simulink model "BMS_MCU_CODE"  (R2025b)
settings: Solver=FixedStepAuto  StartTime=0.0  StopTime=10  MaxStep=.01  RelTol=1e-3  EnableMultiTasking=on
PreLoadFcn:
  | %setup_sil;
  | setup_pil;
InitFcn:
  | battery_init;
  | Full_Charge_Volt=4.2; % unit volts
  | Cutoff_Volt=3; % unit volts
  | Delta=.02;
  | ContactorTime=20;
  | ContactorTimeOut=100;
  | High_TempLim=333;
  | Low_TempLim=253;
  | Sensor_Fault_Treshold=.02;
  | CurrentTimeout=1;
  | Allowed_Delta=.04;
  | Bal_On_Time=30;
  | Bal_Off_Time=5;
  | BalNotAct_Time=10;
values from neighbouring files (symbols this model uses):
  bonka_R0 = [ ... (first row only)    [battery_init.m]
  bonka_SOC = [0, 0.1, 0.2, 0.3, 0.4, 0.5, 0.6, 0.7, 0.8, 0.9, 1.0]    [battery_init.m]
  bonka_T = [263.15, 273.15, 298.15, 313.15, 328.15]    [battery_init.m]
  Capacity = 5.200    (= 5.2)    [MCU.m]
  Charge_Rate = 1    [battery_init.m]
  Discharge_Rate = -1    [battery_init.m]
undefined symbols (not defined in the file or in its folder): DiscIntNeverNeededParam
libraries: simulink x30
settings Model: DataDictionary=Needed_Buses.sldd  STM32="{\"DigitalPortWrite\":[{\"ID\":\"MCU_CODE:12\"},{\"ID\":\"MCU_CODE_Copy:132\"},{\"ID\":\"BMS_PIL_Wrapper:132\"}],\"DigitalPortRead\":[{\"ID\":\"MCU_CODE_Copy:131\"},{\"ID\":\"BMS_PIL_Wrapper:131\"}]}"  SILPILSystemUnderTest=refmodels  CodeVerificationMode=processor-in-the-loop (pil)  Creator=Odonata-KJ  LastModifiedBy=Odonata-KJ
settings DataIOCC: SaveOutput=off  SaveTime=off
settings OptimizationCC: DefaultParameterBehavior=Inlined  EnhancedBackFolding=on  PassReuseOutputArgsAs=Individual arguments  ZeroExternalMemoryAtStartup=off  ZeroInternalMemoryAtStartup=off  MaxStackSize=512  OptimizeBlockOrder=speed  DifferentSizesBufferReuse=on  OptimizationCustomize=off  EfficientTunableParamExpr=on
settings DebuggingCC: ParameterTunabilityLossMsg=error  SFUnexpectedBacktrackingDiag=warning  SFNoUnconditionalDefaultTransitionDiag=warning  UnderSpecifiedDimensionMsg=warning
settings HardwareCC: ProdBitPerPointer=32.0  ProdBitPerSizeT=32.0  ProdBitPerPtrDiffT=32.0  ProdLargestAtomicInteger=Long  ProdLargestAtomicFloat=Double  ProdWordSize=32.0  ProdLongLongMode=on  ProdHWDeviceType=ARM Compatible->ARM Cortex-M  TargetLargestAtomicInteger=Long  TargetLargestAtomicFloat=Double  TargetIntDivRoundTo=Zero  TargetEndianess=LittleEndian  TargetHWDeviceType=ARM Compatible->ARM Cortex-M
settings SFSimCC: MATLABDynamicMemAlloc=off
settings RTWCC: SystemTargetFile=ert.tlc  HardwareBoard=STM32F4xx Based  TemplateMakefile=ert_default_tmf  GenerateReport=on  Toolchain=GNU Tools for ARM Embedded Processors  BuildConfiguration=Debug  LaunchReport=on  PortableWordSizes=on  Description=Embedded Coder
settings CodeAppCC: ForceParamTrailComments=on  IgnoreCustomStorageClasses=off  OperatorAnnotations=on  SimulinkDataObjDesc=on  SFDataObjDesc=on  InsertBlockDesc=on  EnableCustomComments=on
settings ERTTargetCC: ExtModeTransport=3.0  ExtModeStaticAlloc=on  ExtModeStaticAllocSize=2048.0  ExtModeMexFile=ext_xcp  ExtModeIntrfLevel=Level2 - Open  TargetLangStandard=C99 (ISO)

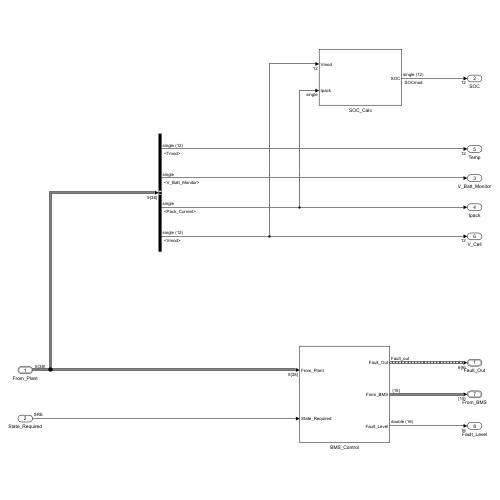
[thumbnail: Simulink's stored preview of the top-level diagram]
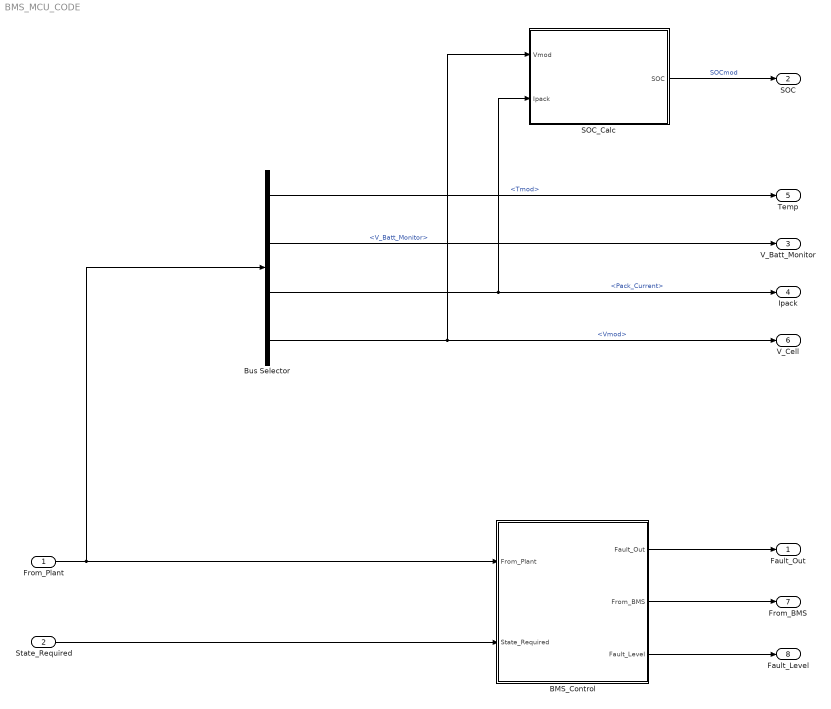
== system BMS_MCU_CODE ==
  From_Plant : Inport  OutDataTypeStr=Bus: From_Plant
  State_Required : Inport  Port=2  OutDataTypeStr=Enum: SRE
  BMS_Control : Subsystem
  Bus Selector : BusSelector  OutputSignals=Tmod,V_Batt_Monitor,Pack_Current,Vmod
  SOC_Calc : Subsystem
  Fault_Out : Outport  OutDataTypeStr=Bus: Fault_out
  SOC : Outport  Port=2
  V_Batt_Monitor : Outport  Port=3
  Ipack : Outport  Port=4
  Temp : Outport  Port=5
  V_Cell : Outport  Port=6
  From_BMS : Outport  Port=7  OutDataTypeStr=Bus: From_BMS
  Fault_Level : Outport  Port=8
  wires:
  From_Plant/1 -> Bus Selector/1, BMS_Control/1(From_Plant)
  BMS_Control/1(Fault_Out) -> Fault_Out/1
  SOC_Calc/1(SOC) -> SOC/1  "SOCmod"
  Bus Selector/1 -> Temp/1  "<Tmod>"
  Bus Selector/3 -> SOC_Calc/2(Ipack), Ipack/1  "<Pack_Current>"
  Bus Selector/4 -> SOC_Calc/1(Vmod), V_Cell/1  "<Vmod>"
  State_Required/1 -> BMS_Control/2(State_Required)
  BMS_Control/2(From_BMS) -> From_BMS/1
  BMS_Control/3(Fault_Level) -> Fault_Level/1
  Bus Selector/2 -> V_Batt_Monitor/1  "<V_Batt_Monitor>"

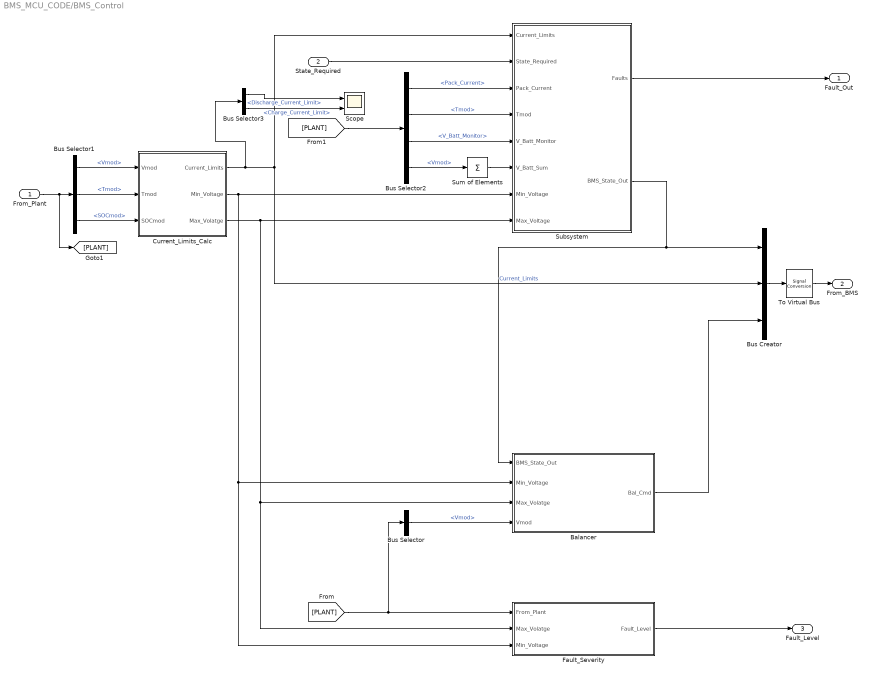
== system BMS_MCU_CODE/BMS_Control ==
  From_Plant : Inport
  State_Required : Inport  Port=2
  Balancer : Subsystem
  Bus Creator : BusCreator  Inputs=3
  Bus Selector : BusSelector  OutputSignals=Vmod
  Bus Selector1 : BusSelector  OutputSignals=Vmod,Tmod,SOCmod
  Bus Selector2 : BusSelector  OutputSignals=Pack_Current,Tmod,V_Batt_Monitor,Vmod
  Bus Selector3 : BusSelector  OutputSignals=Discharge_Current_Limit,Charge_Current_Limit
  Current_Limits_Calc : Subsystem
  Fault_Severity : Subsystem
  Scope : Scope  NumInputPorts=2
  Subsystem : Subsystem
  Sum of Elements : Sum  Inputs=+
  To Virtual Bus : SignalConversion  ConversionOutput=Virtual bus  OverrideOpt=off
  Fault_Out : Outport
  From_BMS : Outport  Port=2  OutDataTypeStr=Bus: From_BMS
  Fault_Level : Outport  Port=3
  wires:
  Bus Selector1/2 -> Current_Limits_Calc/2(Tmod)  "<Tmod>"
  Subsystem/1(Faults) -> Fault_Out/1
  [PLANT] -> Bus Selector2/1
  State_Required/1 -> Subsystem/2(State_Required)
  Current_Limits_Calc/1(Current_Limits) -> Bus Selector3/1, Bus Creator/2, Subsystem/1(Current_Limits)  "Current_Limits"
  Bus Selector1/1 -> Current_Limits_Calc/1(Vmod)  "<Vmod>"
  From_Plant/1 -> Bus Selector1/1, [PLANT]
  Bus Selector2/1 -> Subsystem/3(Pack_Current)  "<Pack_Current>"
  Bus Selector2/2 -> Subsystem/4(Tmod)  "<Tmod>"
  Bus Selector2/3 -> Subsystem/5(V_Batt_Monitor)  "<V_Batt_Monitor>"
  Bus Selector1/3 -> Current_Limits_Calc/3(SOCmod)  "<SOCmod>"
  Bus Creator/1 -> To Virtual Bus/1
  [PLANT] -> Bus Selector/1, Fault_Severity/1(From_Plant)
  Current_Limits_Calc/2(Min_Voltage) -> Fault_Severity/3(Min_Voltage), Balancer/2(Min_Voltage), Subsystem/7(Min_Voltage)
  Bus Selector/1 -> Balancer/4(Vmod)  "<Vmod>"
  Current_Limits_Calc/3(Max_Volatge) -> Fault_Severity/2(Max_Volatge), Balancer/3(Max_Volatge), Subsystem/8(Max_Voltage)
  Balancer/1(Bal_Cmd) -> Bus Creator/3
  Sum of Elements/1 -> Subsystem/6(V_Batt_Sum)
  Bus Selector2/4 -> Sum of Elements/1  "<Vmod>"
  To Virtual Bus/1 -> From_BMS/1
  Subsystem/2(BMS_State_Out) -> Bus Creator/1, Balancer/1(BMS_State_Out)
  Fault_Severity/1(Fault_Level) -> Fault_Level/1
  Bus Selector3/1 -> Scope/1  "<Discharge_Current_Limit>"
  Bus Selector3/2 -> Scope/2  "<Charge_Current_Limit>"

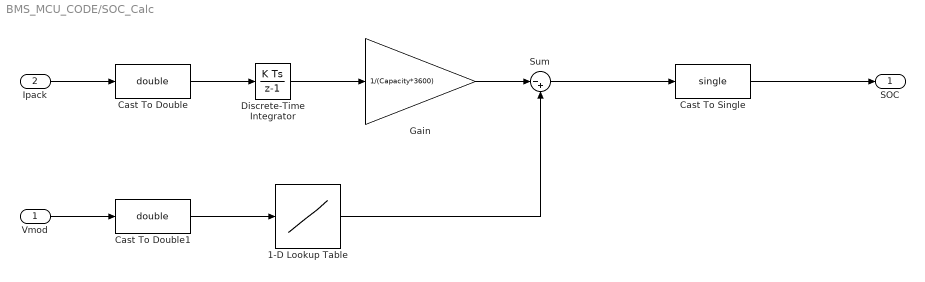
== system BMS_MCU_CODE/SOC_Calc ==
  Vmod : Inport
  Ipack : Inport  Port=2  OutDataTypeStr=single
  1-D Lookup Table : Lookup_n-D  NumberOfTableDimensions=1  BreakpointsForDimension1=[3.0, 3.4, 3.6, 3.7, 3.8, 3.9, 4.0, 4.1, 4.2]  Table=[0.0, 0.1, 0.25, 0.45, 0.62, 0.78, 0.88, 0.95, 1.0]  InternalRulePriority=Speed  RndMeth=Simplest
  Cast To Double : DataTypeConversion  OutDataTypeStr=double  SaturateOnIntegerOverflow=off  RndMeth=Floor
  Cast To Double1 : DataTypeConversion  OutDataTypeStr=double  SaturateOnIntegerOverflow=off  RndMeth=Floor
  Cast To Single : DataTypeConversion  OutDataTypeStr=single  SaturateOnIntegerOverflow=off  RndMeth=Floor
  Discrete-Time Integrator : DiscreteIntegrator  SampleTime=.001  ICPrevOutput=DiscIntNeverNeededParam  ICPrevScaledInput=DiscIntNeverNeededParam
  Gain : Gain  Gain=1/(Capacity*3600)
  Sum : Sum  Inputs=|-+
  SOC : Outport
  wires:
  Cast To Double1/1 -> 1-D Lookup Table/1
  Cast To Single/1 -> SOC/1
  Sum/1 -> Cast To Single/1
  1-D Lookup Table/1 -> Sum/2
  Vmod/1 -> Cast To Double1/1
  Gain/1 -> Sum/1
  Discrete-Time Integrator/1 -> Gain/1
  Ipack/1 -> Cast To Double/1
  Cast To Double/1 -> Discrete-Time Integrator/1

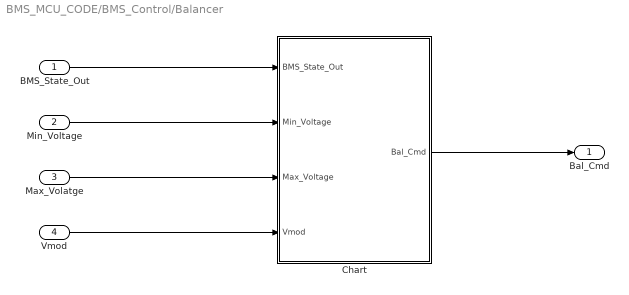
== system BMS_MCU_CODE/BMS_Control/Balancer ==
  BMS_State_Out : Inport
  Min_Voltage : Inport  Port=2
  Max_Volatge : Inport  Port=3
  Vmod : Inport  Port=4
  Chart : Stateflow chart  TreatAsAtomicUnit=on
  Bal_Cmd : Outport
  wires:
  BMS_State_Out/1 -> Chart/1(BMS_State_Out)
  Min_Voltage/1 -> Chart/2(Min_Voltage)
  Vmod/1 -> Chart/4(Vmod)
  Max_Volatge/1 -> Chart/3(Max_Voltage)
  Chart/1(Bal_Cmd) -> Bal_Cmd/1

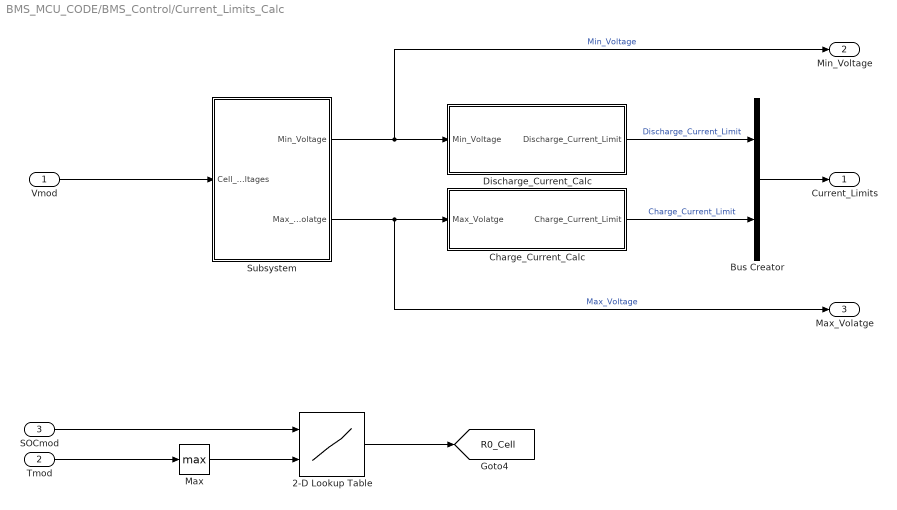
== system BMS_MCU_CODE/BMS_Control/Current_Limits_Calc ==
  Vmod : Inport
  Tmod : Inport  Port=2
  SOCmod : Inport  Port=3
  2-D Lookup Table : Lookup_n-D  BreakpointsForDimension1=bonka_SOC  BreakpointsForDimension2=bonka_T  Table=bonka_R0  InternalRulePriority=Speed  RndMeth=Simplest
      settings: InputPortMap=u0,u1
  Bus Creator : BusCreator  Inputs=2
  Charge_Current_Calc : Subsystem
  Discharge_Current_Calc : Subsystem
  Max : MinMax  Function=max
  Subsystem : Subsystem
  Current_Limits : Outport
  Min_Voltage : Outport  Port=2
  Max_Volatge : Outport  Port=3
  tag scope: R0_Cell=global
  wires:
  Max/1 -> 2-D Lookup Table/2
  2-D Lookup Table/1 -> [R0_Cell]
  SOCmod/1 -> 2-D Lookup Table/1
  Bus Creator/1 -> Current_Limits/1
  Charge_Current_Calc/1(Charge_Current_Limit) -> Bus Creator/2  "Charge_Current_Limit"
  Discharge_Current_Calc/1(Discharge_Current_Limit) -> Bus Creator/1  "Discharge_Current_Limit"
  Subsystem/2(Max_Volatge) -> Max_Volatge/1, Charge_Current_Calc/1(Max_Volatge)  "Max_Voltage"
  Tmod/1 -> Max/1
  Subsystem/1(Min_Voltage) -> Min_Voltage/1, Discharge_Current_Calc/1(Min_Voltage)  "Min_Voltage"
  Vmod/1 -> Subsystem/1(Cell_Voltages)

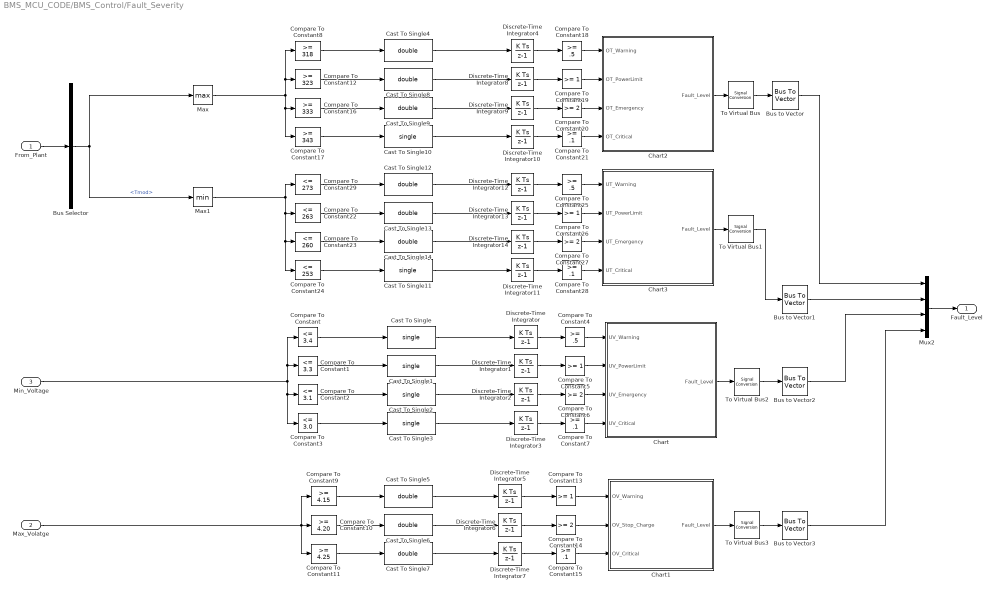
== system BMS_MCU_CODE/BMS_Control/Fault_Severity ==
  From_Plant : Inport
  Max_Volatge : Inport  Port=2
  Min_Voltage : Inport  Port=3
  Bus Selector : BusSelector  OutputSignals=Tmod
  Bus to Vector{,1..3} (4 alike) : BusToVector
  Cast To Single{,1..3,10..11} (6 alike) : DataTypeConversion  OutDataTypeStr=single  SaturateOnIntegerOverflow=off  RndMeth=Floor
  Cast To Single{4..9,12..14} (9 alike) : DataTypeConversion  OutDataTypeStr=double  SaturateOnIntegerOverflow=off  RndMeth=Floor
  Chart : Stateflow chart  TreatAsAtomicUnit=on
  Chart1 : Stateflow chart  TreatAsAtomicUnit=on
  Chart2 : Stateflow chart  TreatAsAtomicUnit=on
  Chart3 : Stateflow chart  TreatAsAtomicUnit=on
  Compare To Constant : simulink/Logic and Bit Operations/Compare To Constant  relop=<=  const=3.4  OutDataTypeStr=boolean
  Compare To Constant1 : simulink/Logic and Bit Operations/Compare To Constant  relop=<=  const=3.3  OutDataTypeStr=boolean
  Compare To Constant10 : simulink/Logic and Bit Operations/Compare To Constant  relop=>=  const=4.20  OutDataTypeStr=boolean
  Compare To Constant11 : simulink/Logic and Bit Operations/Compare To Constant  relop=>=  const=4.25  OutDataTypeStr=boolean
  Compare To Constant12 : simulink/Logic and Bit Operations/Compare To Constant  relop=>=  const=323  OutDataTypeStr=boolean
  Compare To Constant{5,13,19,26} (4 alike) : simulink/Logic and Bit Operations/Compare To Constant  relop=>=  const=1  OutDataTypeStr=boolean
  Compare To Constant{6,14,20,27} (4 alike) : simulink/Logic and Bit Operations/Compare To Constant  relop=>=  const=2  OutDataTypeStr=boolean
  Compare To Constant{7,15,21,28} (4 alike) : simulink/Logic and Bit Operations/Compare To Constant  relop=>=  const=.1  OutDataTypeStr=boolean
  Compare To Constant16 : simulink/Logic and Bit Operations/Compare To Constant  relop=>=  const=333  OutDataTypeStr=boolean
  Compare To Constant17 : simulink/Logic and Bit Operations/Compare To Constant  relop=>=  const=343  OutDataTypeStr=boolean
  Compare To Constant18 : simulink/Logic and Bit Operations/Compare To Constant  relop=>=  const=.5  OutDataTypeStr=boolean
  Compare To Constant2 : simulink/Logic and Bit Operations/Compare To Constant  relop=<=  const=3.1  OutDataTypeStr=boolean
  Compare To Constant22 : simulink/Logic and Bit Operations/Compare To Constant  relop=<=  const=263  OutDataTypeStr=boolean
  Compare To Constant23 : simulink/Logic and Bit Operations/Compare To Constant  relop=<=  const=260  OutDataTypeStr=boolean
  Compare To Constant24 : simulink/Logic and Bit Operations/Compare To Constant  relop=<=  const=253  OutDataTypeStr=boolean
  Compare To Constant25 : simulink/Logic and Bit Operations/Compare To Constant  relop=>=  const=.5  OutDataTypeStr=boolean
  Compare To Constant29 : simulink/Logic and Bit Operations/Compare To Constant  relop=<=  const=273  OutDataTypeStr=boolean
  Compare To Constant3 : simulink/Logic and Bit Operations/Compare To Constant  relop=<=  const=3.0  OutDataTypeStr=boolean
  Compare To Constant4 : simulink/Logic and Bit Operations/Compare To Constant  relop=>=  const=.5  OutDataTypeStr=boolean
  Compare To Constant8 : simulink/Logic and Bit Operations/Compare To Constant  relop=>=  const=318  OutDataTypeStr=boolean
  Compare To Constant9 : simulink/Logic and Bit Operations/Compare To Constant  relop=>=  const=4.15  OutDataTypeStr=boolean
  Discrete-Time Integrator{,1..14} (15 alike) : DiscreteIntegrator  SampleTime=.001  ICPrevOutput=DiscIntNeverNeededParam  ICPrevScaledInput=DiscIntNeverNeededParam
  Max : MinMax  Function=max
  Max1 : MinMax
  Mux2 : Mux
  To Virtual Bus{,1..3} (4 alike) : SignalConversion  ConversionOutput=Virtual bus  OverrideOpt=off
  Fault_Level : Outport
  wires:
  From_Plant/1 -> Bus Selector/1
  Min_Voltage/1 -> Compare To Constant3/1, Compare To Constant2/1, Compare To Constant/1, Compare To Constant1/1
  Compare To Constant/1 -> Cast To Single/1
  Compare To Constant1/1 -> Cast To Single1/1
  Compare To Constant2/1 -> Cast To Single2/1
  Compare To Constant3/1 -> Cast To Single3/1
  Cast To Single/1 -> Discrete-Time Integrator/1
  Cast To Single1/1 -> Discrete-Time Integrator1/1
  Cast To Single2/1 -> Discrete-Time Integrator2/1
  Discrete-Time Integrator/1 -> Compare To Constant4/1
  Discrete-Time Integrator1/1 -> Compare To Constant5/1
  Discrete-Time Integrator2/1 -> Compare To Constant6/1
  Discrete-Time Integrator3/1 -> Compare To Constant7/1
  Cast To Single3/1 -> Discrete-Time Integrator3/1
  Compare To Constant4/1 -> Chart/1(UV_Warning)
  Compare To Constant5/1 -> Chart/2(UV_PowerLimit)
  Compare To Constant6/1 -> Chart/3(UV_Emergency)
  Compare To Constant7/1 -> Chart/4(UV_Critical)
  Compare To Constant14/1 -> Chart1/2(OV_Stop_Charge)
  Max_Volatge/1 -> Compare To Constant9/1, Compare To Constant11/1, Compare To Constant10/1
  Discrete-Time Integrator6/1 -> Compare To Constant14/1
  Discrete-Time Integrator5/1 -> Compare To Constant13/1
  Compare To Constant13/1 -> Chart1/1(OV_Warning)
  Cast To Single6/1 -> Discrete-Time Integrator6/1
  Cast To Single7/1 -> Discrete-Time Integrator7/1
  Compare To Constant10/1 -> Cast To Single6/1
  Compare To Constant9/1 -> Cast To Single5/1
  Compare To Constant15/1 -> Chart1/3(OV_Critical)
  Compare To Constant11/1 -> Cast To Single7/1
  Discrete-Time Integrator7/1 -> Compare To Constant15/1
  Cast To Single5/1 -> Discrete-Time Integrator5/1
  Bus Selector/1 -> Max/1, Max1/1  "<Tmod>"
  Discrete-Time Integrator4/1 -> Compare To Constant18/1
  Compare To Constant20/1 -> Chart2/3(OT_Emergency)
  Max/1 -> Compare To Constant8/1, Compare To Constant12/1, Compare To Constant17/1, Compare To Constant16/1
  Discrete-Time Integrator9/1 -> Compare To Constant20/1
  Discrete-Time Integrator8/1 -> Compare To Constant19/1
  Compare To Constant19/1 -> Chart2/2(OT_PowerLimit)
  Cast To Single9/1 -> Discrete-Time Integrator9/1
  Cast To Single10/1 -> Discrete-Time Integrator10/1
  Cast To Single4/1 -> Discrete-Time Integrator4/1
  Compare To Constant16/1 -> Cast To Single9/1
  Compare To Constant12/1 -> Cast To Single8/1
  Compare To Constant21/1 -> Chart2/4(OT_Critical)
  Compare To Constant8/1 -> Cast To Single4/1
  Compare To Constant18/1 -> Chart2/1(OT_Warning)
  Compare To Constant17/1 -> Cast To Single10/1
  Discrete-Time Integrator10/1 -> Compare To Constant21/1
  Cast To Single8/1 -> Discrete-Time Integrator8/1
  Compare To Constant25/1 -> Chart3/1(UT_Warning)
  Max1/1 -> Compare To Constant22/1, Compare To Constant23/1, Compare To Constant24/1, Compare To Constant29/1
  Compare To Constant24/1 -> Cast To Single11/1
  Compare To Constant22/1 -> Cast To Single13/1
  Cast To Single13/1 -> Discrete-Time Integrator13/1
  Compare To Constant29/1 -> Cast To Single12/1
  Discrete-Time Integrator11/1 -> Compare To Constant28/1
  Compare To Constant23/1 -> Cast To Single14/1
  Discrete-Time Integrator14/1 -> Compare To Constant27/1
  Cast To Single14/1 -> Discrete-Time Integrator14/1
  Compare To Constant26/1 -> Chart3/2(UT_PowerLimit)
  Compare To Constant28/1 -> Chart3/4(UT_Critical)
  Cast To Single12/1 -> Discrete-Time Integrator12/1
  Discrete-Time Integrator13/1 -> Compare To Constant26/1
  Discrete-Time Integrator12/1 -> Compare To Constant25/1
  Compare To Constant27/1 -> Chart3/3(UT_Emergency)
  Cast To Single11/1 -> Discrete-Time Integrator11/1
  Chart2/1(Fault_Level) -> To Virtual Bus/1
  Chart3/1(Fault_Level) -> To Virtual Bus1/1
  Chart/1(Fault_Level) -> To Virtual Bus2/1
  Chart1/1(Fault_Level) -> To Virtual Bus3/1
  Mux2/1 -> Fault_Level/1
  Bus to Vector/1 -> Mux2/1
  Bus to Vector1/1 -> Mux2/2
  Bus to Vector2/1 -> Mux2/3
  Bus to Vector3/1 -> Mux2/4
  To Virtual Bus/1 -> Bus to Vector/1
  To Virtual Bus1/1 -> Bus to Vector1/1
  To Virtual Bus2/1 -> Bus to Vector2/1
  To Virtual Bus3/1 -> Bus to Vector3/1

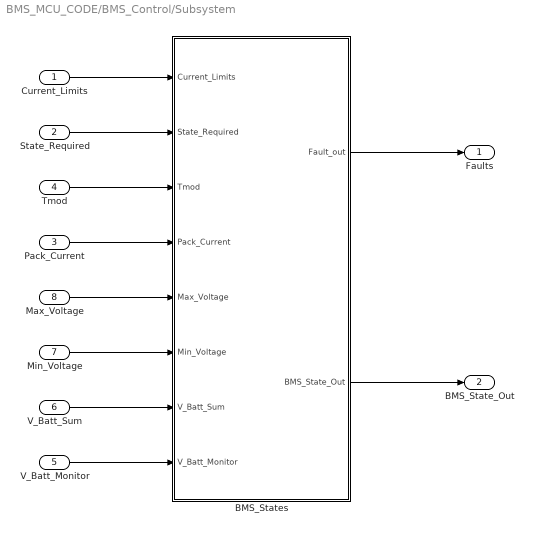
== system BMS_MCU_CODE/BMS_Control/Subsystem ==
  Current_Limits : Inport
  State_Required : Inport  Port=2
  Pack_Current : Inport  Port=3  OutDataTypeStr=single
  Tmod : Inport  Port=4
  V_Batt_Monitor : Inport  Port=5
  V_Batt_Sum : Inport  Port=6  OutDataTypeStr=single
  Min_Voltage : Inport  Port=7
  Max_Voltage : Inport  Port=8
  BMS_States : Stateflow chart  TreatAsAtomicUnit=on
      settings: PortSchema="{\"entries\":[{\"content\":{\"sides\":[{\"content\":{\"connectorIds\":[\"In1\",\"In5\",\"In2\",\"In3\",\"In6\",\"In7\",\"In4\",\"In8\"]},\"type\":\"ConnectorPlacement.EquallySpacedRectSide\",\"uuid\":\"75752650-a65f-4df2-8429-36d8f2b8ac99\"},{\"content\":{\"connectorIds\":[\"Out1\",\"Out2\"],\"side\":\"RIGHT\"},\"type\":\"ConnectorPlacement.EquallySpacedRectSide\",\"uuid\":\"5c64a1aa-fdb2-4c0c-b2ff-5c47ddc01ea2\"},{\"content\":{\"side\":\"TOP\"},\"type\":\"ConnectorPlacement.EquallySpacedRectSide\",\"uuid\":\"c92e07e0-a1c3-44d4-87a0-5a0cb4ce56f3\"}]},\"type\":\"ConnectorPlacement.EquallySpacedConnector\",\"uuid\":\"9d97857d-a16c-4ff3-995b-4c10703be4f7\"}],\"packageUris\":[\"http://schema.mathworks.com/mf0/Connector/R2020b\"],\"version\":\"1.0\"}"
  Faults : Outport
  BMS_State_Out : Outport  Port=2
  wires:
  BMS_States/2(BMS_State_Out) -> BMS_State_Out/1
  BMS_States/1(Fault_out) -> Faults/1
  Current_Limits/1 -> BMS_States/1(Current_Limits)
  State_Required/1 -> BMS_States/5(State_Required)
  Min_Voltage/1 -> BMS_States/7(Min_Voltage)
  Max_Voltage/1 -> BMS_States/6(Max_Voltage)
  V_Batt_Sum/1 -> BMS_States/4(V_Batt_Sum)
  Pack_Current/1 -> BMS_States/3(Pack_Current)
  Tmod/1 -> BMS_States/2(Tmod)
  V_Batt_Monitor/1 -> BMS_States/8(V_Batt_Monitor)

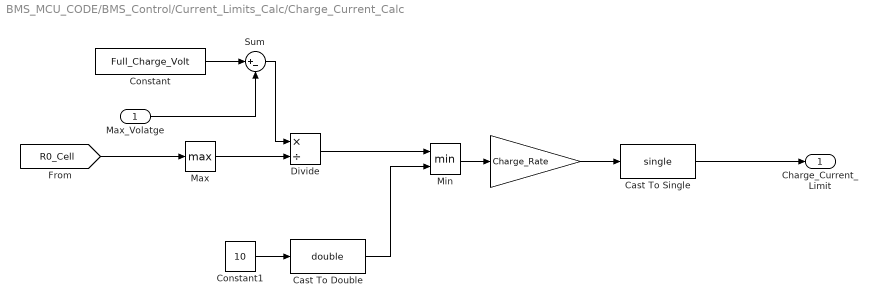
== system BMS_MCU_CODE/BMS_Control/Current_Limits_Calc/Charge_Current_Calc ==
  Max_Volatge : Inport
  " " : Gain  Gain=Charge_Rate
  Cast To Double : DataTypeConversion  OutDataTypeStr=double  SaturateOnIntegerOverflow=off  RndMeth=Floor
  Cast To Single : DataTypeConversion  OutDataTypeStr=single  SaturateOnIntegerOverflow=off  RndMeth=Floor
  Constant : Constant  Value=Full_Charge_Volt
  Constant1 : Constant  Value=10
  Divide : Product  Inputs=*/
  Max : MinMax  Function=max
  Min : MinMax  Inputs=2
  Sum : Sum  Inputs=|+-
  Charge_Current_Limit : Outport
  wires:
  Max/1 -> Divide/2
  " "/1 -> Cast To Single/1
  Cast To Single/1 -> Charge_Current_Limit/1
  Divide/1 -> Min/1
  [R0_Cell] -> Max/1
  Sum/1 -> Divide/1
  Max_Volatge/1 -> Sum/2
  Constant/1 -> Sum/1
  Constant1/1 -> Cast To Double/1
  Min/1 -> " "/1
  Cast To Double/1 -> Min/2

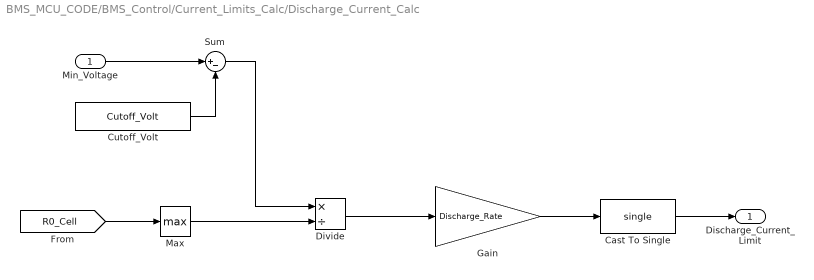
== system BMS_MCU_CODE/BMS_Control/Current_Limits_Calc/Discharge_Current_Calc ==
  Min_Voltage : Inport
  Cast To Single : DataTypeConversion  OutDataTypeStr=single  SaturateOnIntegerOverflow=off  RndMeth=Floor
  Cutoff_Volt : Constant  Value=Cutoff_Volt
  Divide : Product  Inputs=*/
  Gain : Gain  Gain=Discharge_Rate
  Max : MinMax  Function=max
  Sum : Sum  Inputs=|+-
  Discharge_Current_Limit : Outport
  wires:
  [R0_Cell] -> Max/1
  Gain/1 -> Cast To Single/1
  Cast To Single/1 -> Discharge_Current_Limit/1
  Divide/1 -> Gain/1
  Max/1 -> Divide/2
  Sum/1 -> Divide/1
  Cutoff_Volt/1 -> Sum/2
  Min_Voltage/1 -> Sum/1

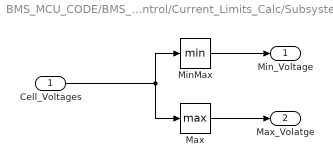
== system BMS_MCU_CODE/BMS_Control/Current_Limits_Calc/Subsystem ==
  Cell_Voltages : Inport
  Max : MinMax  Function=max
  MinMax : MinMax
  Min_Voltage : Outport
  Max_Volatge : Outport  Port=2
  wires:
  Max/1 -> Max_Volatge/1
  MinMax/1 -> Min_Voltage/1
  Cell_Voltages/1 -> MinMax/1, Max/1

== stateflow chart BMS_MCU_CODE/BMS_Control/Fault_Severity/Chart1 ==
  state UV_Fault_Severity
    during:
    if OV_Critical
    Fault_Level.OV = 3;
    elseif OV_Stop_Charge
    Fault_Level.OV = 2;
    elseif OV_Warning
    Fault_Level.OV= 1;
    else
    Fault_Level.OV = 0;
    end
  (default) -> UV_Fault_Severity
  data: OV_Warning input boolean; OV_Stop_Charge input boolean; OV_Critical input boolean; Fault_Level output Bus: Fault_Level

== stateflow chart BMS_MCU_CODE/BMS_Control/Balancer/Chart ==
  state Balancing_Off
    en:
    Bal_Cmd(:,:)= false;
    en, du:
    DeltaCellVolt=Max_Voltage-Min_Voltage;
  state Balancing_On
    en, du:
    DeltaCellVolt=Max_Voltage-Min_Voltage;
    state Balance_Active
      en, du:
      Bal_Cmd=((Vmod-Min_Voltage)> Allowed_Delta/2)';
      flgBalCompl=all(~Bal_Cmd);
    state Balance_Not_Active
    (default) -> Balance_Active
    Balance_Not_Active -> Balance_Active [order 1] : [after(BalNotAct_Time, sec) &&...
        |  DeltaCellVolt> Allowed_Delta]
    Balance_Active -> Balance_Not_Active : [flgBalCompl]
  (default) -> Balancing_Off : {flgBalCompl=true}
  Balancing_Off -> Balancing_On : [flgBalInt &&...
      | BMS_State_Out==BMS_State.Charging &&...
      | after(Bal_Off_Time, sec) &&...
      | DeltaCellVolt> Allowed_Delta]
  Balancing_On -> Balancing_Off : [BMS_State_Out==BMS_State.Flying]
  Balance_Not_Active -> Balancing_Off [order 2] : [after(Bal_On_Time, sec)]
  data: BMS_State_Out input; Min_Voltage input single; Max_Voltage input single; Bal_Cmd output boolean size=[1 12]; Allowed_Delta parameter single; DeltaCellVolt local single; Bal_On_Time parameter single; Bal_Off_Time parameter single; BalNotAct_Time parameter single; Vmod input single; flgBalCompl local boolean =false; flgBalInt local =true

== stateflow chart BMS_MCU_CODE/BMS_Control/Fault_Severity/Chart ==
  state UV_Fault_Severity
    during:
    if UV_Critical
    Fault_Level.UV = 4;
    elseif UV_Emergency
    Fault_Level.UV = 3;
    elseif UV_PowerLimit
    Fault_Level.UV = 2;
    elseif UV_Warning
    Fault_Level.UV = 1;
    else
    Fault_Level.UV = 0;
    end
  (default) -> UV_Fault_Severity
  data: UV_Warning input boolean; UV_PowerLimit input boolean; UV_Emergency input boolean; UV_Critical input boolean; Fault_Level output Bus: Fault_Level

== stateflow chart BMS_MCU_CODE/BMS_Control/Subsystem/BMS_States ==
  state Fault_Monitoring [parallel]
    settings: executionOrder=2
    state Monitor_CurrentLim [parallel]
      settings: executionOrder=1
      state No_CurrentLim_Fault
      state Wait
      state OC_Fault
        en:
        FaultPresent=true;
        Fault_out.OC=true;
      (default) -> No_CurrentLim_Fault : {FaultPresent=false;
          |  Fault_out.OC=false;}
      No_CurrentLim_Fault -> Wait : [(Pack_Current< Current_Limits.Discharge_Current_Limit) || ...
          | (Pack_Current> Current_Limits.Charge_Current_Limit)]
      Wait -> No_CurrentLim_Fault [order 2] : [(Pack_Current >= Current_Limits.Discharge_Current_Limit) && ...
          | (Pack_Current <= Current_Limits.Charge_Current_Limit)]
      Wait -> OC_Fault [order 1] : [after(CurrentTimeout, sec)]
    state Monitor_CellVolt [parallel]
      settings: executionOrder=3
      state No_OV_UV
        en,du:
        Delta=abs(V_Batt_Sum-V_Batt_Monitor);
      state OV_Fault
        en:
        FaultPresent=true;
        Fault_out.OV=true;
      state UV_Fault
        en:
        FaultPresent=true;
        Fault_out.UV=true;
      state Sensor_Fault
        en:
        FaultPresent=true;
        Fault_out.VoltSensor=true;
      (default) -> No_OV_UV : {FaultPresent=false;
          | Fault_out.VoltSensor=false;
          | Fault_out.UV=false;
          | Fault_out.OV=false;}
      No_OV_UV -> OV_Fault [order 3] : [Max_Voltage>=Full_Charge_Volt]
      No_OV_UV -> (junction 89) [order 2] : [Min_Voltage <= Cutoff_Volt]
      (junction 89) -> UV_Fault
      (junction 173) -> No_OV_UV : [[Min_Voltage > Cutoff_Volt]]
      UV_Fault -> (junction 173)
      No_OV_UV -> Sensor_Fault [order 1] : [Delta>=single(Sensor_Fault_Treshold)]
    state Monitor_CellTemp [parallel]
      settings: executionOrder=2
      state OT_Fault
        en:
        FaultPresent=true;
        Fault_out.OT=true;
      state No_OT_UT
        en, du:
        MaxCellTemp=max(Tmod);
        MinCellTemp=min(Tmod);
      state UT_Fault
        en:
        FaultPresent=true;
        Fault_out.UT=true;
      No_OT_UT -> OT_Fault [order 2] : [MaxCellTemp>=High_TempLim]
      (default) -> No_OT_UT : {FaultPresent=false;
          | Fault_out.OT=false;
          | Fault_out.UT=false;}
      No_OT_UT -> UT_Fault [order 1] : [MinCellTemp<=Low_TempLim]
  state Normal_State [parallel]
    settings: executionOrder=1
    state Idle
      en:
      BMS_State_Out= BMS_State.Standbying
    state Charging
      en:
      BMS_State_Out= BMS_State.Charging
    state Flying
      en:
      BMS_State_Out= BMS_State.Flying
    state Fault
      en,du:
      BMS_State_Out= BMS_State.Fault
    (default) -> Idle
    Idle -> Charging [order 2] : [State_Required==SRE.Charge ]
    Idle -> (junction 51) [order 3] : [FaultPresent]
    (junction 51) -> (junction 52)
    Charging -> Idle [order 1] : [(State_Required~=SRE.Charge)...
        | || (State_Required==SRE.Standby) ]
    Idle -> Flying [order 1] : [State_Required== SRE.Fly]
    Flying -> Idle [order 1] : [(State_Required~=SRE.Fly) ||...
        | (State_Required==SRE.Standby) ]
    (junction 43) -> Charging
    Charging -> (junction 41) [order 2]
    Charging -> Fault [order 3] : [FaultPresent]
    Flying -> (junction 43) [order 2] : [State_Required==SRE.Charge]
    (junction 41) -> Flying : [State_Required== SRE.Fly]
    Flying -> Fault [order 3] : [FaultPresent]
    (junction 52) -> Fault
  data: Current_Limits input Bus: Current_Limits; Tmod input single; Pack_Current input single; V_Batt_Sum input single size=1; State_Required input Enum: SRE; Fault_out output Bus: Fault_out; Max_Voltage input single; Min_Voltage input single; Low_TempLim parameter single; High_TempLim parameter single; Cutoff_Volt parameter single; Full_Charge_Volt parameter single; MaxCellTemp local single; MinCellTemp local single; Delta local single; Sensor_Fault_Treshold parameter double; FaultPresent local boolean; BMS_State_Out output Enum: BMS_State; CurrentTimeout parameter; V_Batt_Monitor input

== stateflow chart BMS_MCU_CODE/BMS_Control/Fault_Severity/Chart2 ==
  state UV_Fault_Severity
    during:
    if OT_Critical
    Fault_Level.OT = 4;
    elseif OT_Emergency
    Fault_Level.OT = 3;
    elseif OT_PowerLimit
    Fault_Level.OT = 2;
    elseif OT_Warning
    Fault_Level.OT = 1;
    else
    Fault_Level.OT = 0;
    end
  (default) -> UV_Fault_Severity
  data: OT_Warning input boolean; OT_PowerLimit input boolean; OT_Emergency input boolean; OT_Critical input boolean; Fault_Level output Bus: Fault_Level

== stateflow chart BMS_MCU_CODE/BMS_Control/Fault_Severity/Chart3 ==
  state UV_Fault_Severity
    during:
    if UT_Critical
    Fault_Level.UT = 4;
    elseif UT_Emergency
    Fault_Level.UT = 3;
    elseif UT_PowerLimit
    Fault_Level.UT = 2;
    elseif UT_Warning
    Fault_Level.UT = 1;
    else
    Fault_Level.UT = 0;
    end
  (default) -> UV_Fault_Severity
  data: UT_Warning input boolean; UT_PowerLimit input boolean; UT_Emergency input boolean; UT_Critical input boolean; Fault_Level output Bus: Fault_Level
